simulink model "DSBSCsimulation"  (R2016a)
settings: Solver=ode3  SolverMode=SingleTasking  StartTime=0.0  StopTime=inf  RelTol=1e-3
libraries: dsparch4 x1
settings Model: Creator=THINKPAD  LastModifiedBy=THINKPAD
settings SolverCC: AutoInsertRateTranBlk=on
settings DataIOCC: LimitDataPoints=on  SaveOutput=off  SignalLogging=off  SaveTime=off
settings DebuggingCC: AlgebraicLoopMsg=error  SingleTaskRateTransMsg=error  AllowSymbolicDim=off

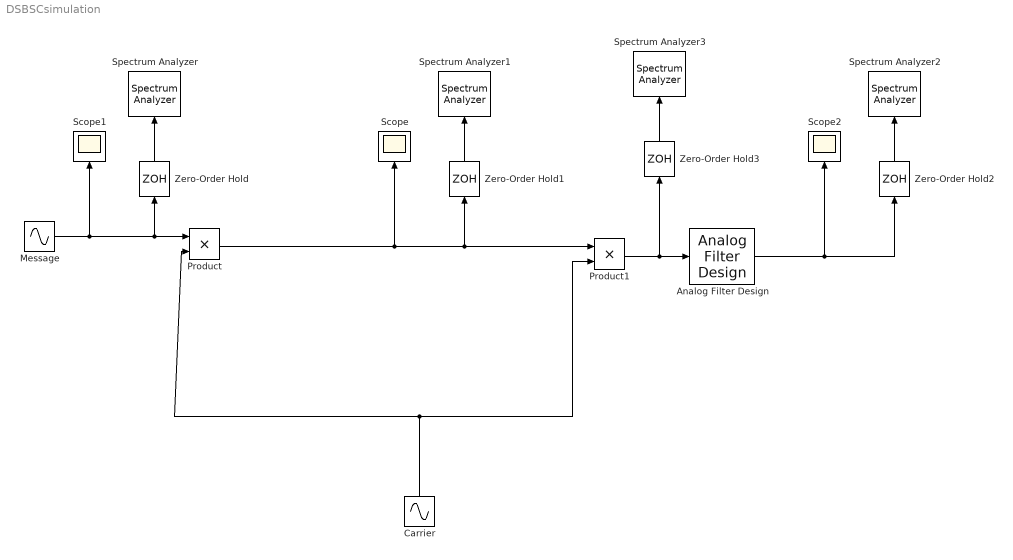
== system DSBSCsimulation ==
  Analog Filter Design : dsparch4/Analog Filter Design  method=Butterworth  filttype=Lowpass  N=8  Wlo=20*pi  Whi=80  Rp=2  Rs=40
  Carrier : Sin  Frequency=100*pi  SampleTime=0
  Message : Sin  Frequency=10*pi  SampleTime=0
  Product : Product
  Product1 : Product
  Scope : Scope
  Scope1 : Scope
  Scope2 : Scope
  Spectrum Analyzer{,1..3} (4 alike) : SpectrumAnalyzer
  Zero-Order Hold : ZeroOrderHold  SampleTime=1/150
  Zero-Order Hold1 : ZeroOrderHold  SampleTime=1/1500
  Zero-Order Hold2 : ZeroOrderHold  SampleTime=1/150
  Zero-Order Hold3 : ZeroOrderHold  SampleTime=1/1500
  wires:
  Carrier/1 -> Product/2, Product1/2
  Product/1 -> Product1/1, Zero-Order Hold1/1, Scope/1
  Zero-Order Hold/1 -> Spectrum Analyzer/1
  Zero-Order Hold1/1 -> Spectrum Analyzer1/1
  Message/1 -> Zero-Order Hold/1, Product/1, Scope1/1
  Analog Filter Design/1 -> Scope2/1, Zero-Order Hold2/1
  Zero-Order Hold2/1 -> Spectrum Analyzer2/1
  Product1/1 -> Analog Filter Design/1, Zero-Order Hold3/1
  Zero-Order Hold3/1 -> Spectrum Analyzer3/1
